simulink model "qbot2_sim_2020b"  (R2020b)
settings: Solver=FixedStepAuto  StartTime=0.0  StopTime=P.t_end  FixedStep=P.dt  RelTol=1e-3
InitFcn:
  | % load_qbot2_sim
StopFcn:
  | if (P.plotsim_flag)
  |     plot_sim(out, P)
  | end
settings Model: Creator=David L Olson  LastModifiedBy=divad

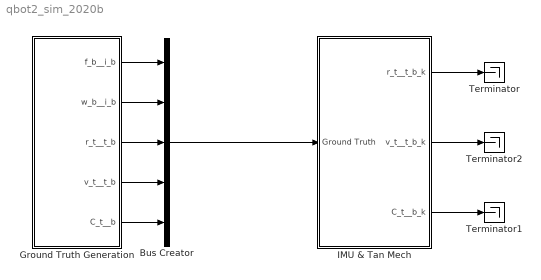
== system qbot2_sim_2020b ==
  Bus Creator : BusCreator  Inputs=5
  Ground Truth Generation : Subsystem
  IMU & Tan Mech : Subsystem
  Terminator : Terminator
  Terminator1 : Terminator
  Terminator2 : Terminator
  wires:
  Ground Truth Generation/1(f_b__i_b) -> Bus Creator/1
  Ground Truth Generation/2(w_b__i_b) -> Bus Creator/2
  Ground Truth Generation/3(r_t__t_b) -> Bus Creator/3
  Ground Truth Generation/4(v_t__t_b) -> Bus Creator/4
  Ground Truth Generation/5(C_t__b) -> Bus Creator/5
  Bus Creator/1 -> IMU & Tan Mech/1(Ground Truth)
  IMU & Tan Mech/1(r_t__t_b_k) -> Terminator/1
  IMU & Tan Mech/2(v_t__t_b_k) -> Terminator2/1
  IMU & Tan Mech/3(C_t__b_k) -> Terminator1/1

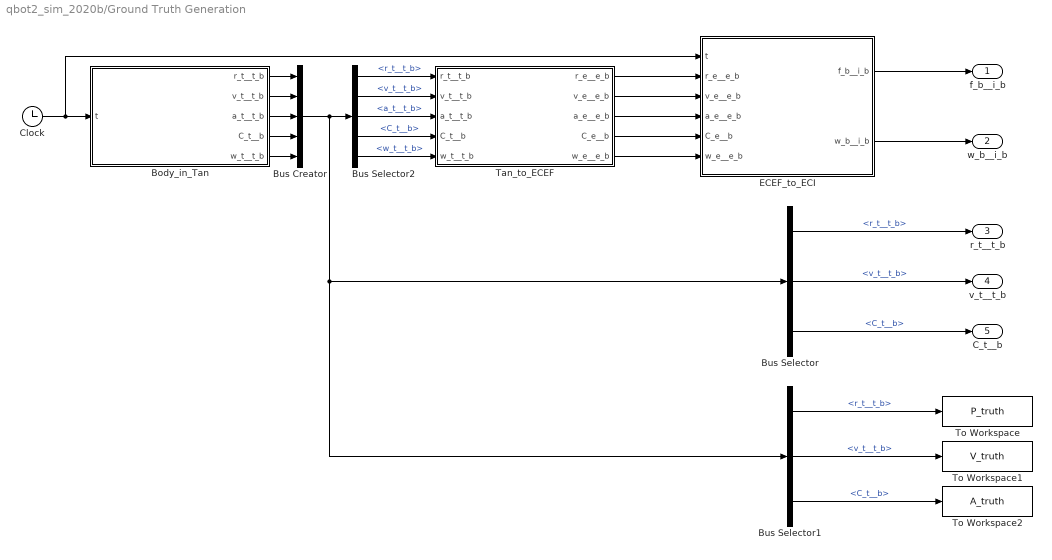
== system qbot2_sim_2020b/Ground Truth Generation ==
  Body_in_Tan : MATLAB Function  TreatAsAtomicUnit=on
  Bus Creator : BusCreator  Inputs=5
  Bus Selector : BusSelector  OutputSignals=r_t__t_b,v_t__t_b,C_t__b
  Bus Selector1 : BusSelector  OutputSignals=r_t__t_b,v_t__t_b,C_t__b
  Bus Selector2 : BusSelector  OutputSignals=r_t__t_b,v_t__t_b,a_t__t_b,C_t__b,w_t__t_b
  Clock : Clock
  ECEF_to_ECI : MATLAB Function  TreatAsAtomicUnit=on
  Tan_to_ECEF : MATLAB Function  TreatAsAtomicUnit=on
  To Workspace : ToWorkspace  VariableName=P_truth  SaveFormat=Timeseries  SampleTime=-1
  To Workspace1 : ToWorkspace  VariableName=V_truth  SaveFormat=Timeseries  SampleTime=-1
  To Workspace2 : ToWorkspace  VariableName=A_truth  SaveFormat=Timeseries  SampleTime=-1
  f_b__i_b : Outport
  w_b__i_b : Outport  Port=2
  r_t__t_b : Outport  Port=3
  v_t__t_b : Outport  Port=4
  C_t__b : Outport  Port=5
  wires:
  Clock/1 -> Body_in_Tan/1(t), ECEF_to_ECI/1(t)
  Tan_to_ECEF/1(r_e__e_b) -> ECEF_to_ECI/2(r_e__e_b)
  Tan_to_ECEF/3(a_e__e_b) -> ECEF_to_ECI/4(a_e__e_b)
  Tan_to_ECEF/2(v_e__e_b) -> ECEF_to_ECI/3(v_e__e_b)
  Tan_to_ECEF/4(C_e__b) -> ECEF_to_ECI/5(C_e__b)
  Tan_to_ECEF/5(w_e__e_b) -> ECEF_to_ECI/6(w_e__e_b)
  ECEF_to_ECI/2(w_b__i_b) -> w_b__i_b/1
  ECEF_to_ECI/1(f_b__i_b) -> f_b__i_b/1
  Body_in_Tan/1(r_t__t_b) -> Bus Creator/1
  Body_in_Tan/2(v_t__t_b) -> Bus Creator/2
  Body_in_Tan/3(a_t__t_b) -> Bus Creator/3
  Body_in_Tan/4(C_t__b) -> Bus Creator/4
  Body_in_Tan/5(w_t__t_b) -> Bus Creator/5
  Bus Creator/1 -> Bus Selector2/1, Bus Selector/1, Bus Selector1/1
  Bus Selector/1 -> r_t__t_b/1  "<r_t__t_b>"
  Bus Selector/2 -> v_t__t_b/1  "<v_t__t_b>"
  Bus Selector/3 -> C_t__b/1  "<C_t__b>"
  Bus Selector2/5 -> Tan_to_ECEF/5(w_t__t_b)  "<w_t__t_b>"
  Bus Selector2/4 -> Tan_to_ECEF/4(C_t__b)  "<C_t__b>"
  Bus Selector2/3 -> Tan_to_ECEF/3(a_t__t_b)  "<a_t__t_b>"
  Bus Selector2/2 -> Tan_to_ECEF/2(v_t__t_b)  "<v_t__t_b>"
  Bus Selector2/1 -> Tan_to_ECEF/1(r_t__t_b)  "<r_t__t_b>"
  Bus Selector1/2 -> To Workspace1/1  "<v_t__t_b>"
  Bus Selector1/1 -> To Workspace/1  "<r_t__t_b>"
  Bus Selector1/3 -> To Workspace2/1  "<C_t__b>"

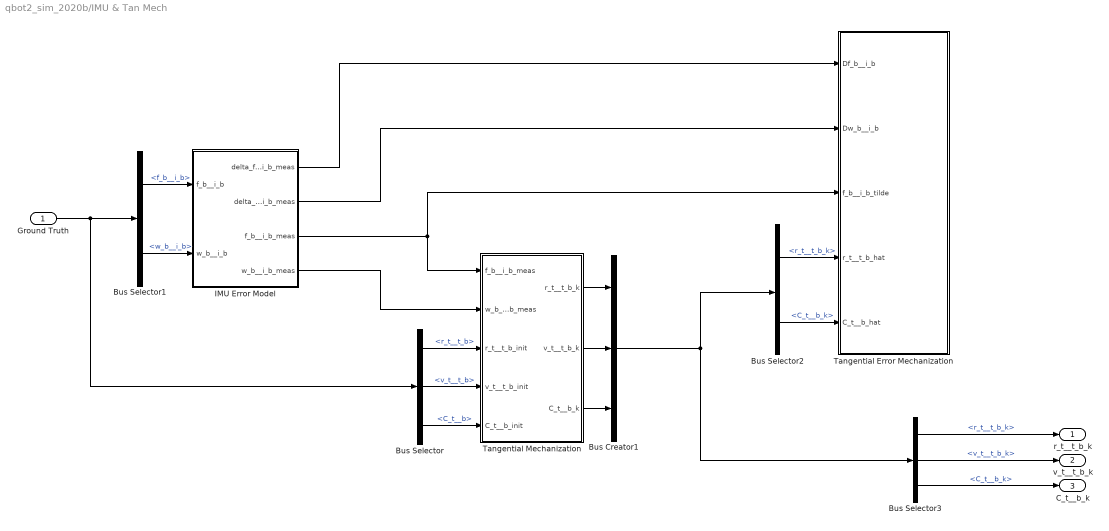
== system qbot2_sim_2020b/IMU & Tan Mech ==
  Ground Truth : Inport
  Bus Creator1 : BusCreator  Inputs=3
  Bus Selector : BusSelector  OutputSignals=r_t__t_b,v_t__t_b,C_t__b
  Bus Selector1 : BusSelector  OutputSignals=f_b__i_b,w_b__i_b
  Bus Selector2 : BusSelector  OutputSignals=r_t__t_b_k,C_t__b_k
  Bus Selector3 : BusSelector  OutputSignals=r_t__t_b_k,v_t__t_b_k,C_t__b_k
  IMU Error Model : Subsystem
  Tangential Error Mechanization : Subsystem
  Tangential Mechanization : Subsystem
  r_t__t_b_k : Outport
  v_t__t_b_k : Outport  Port=2
  C_t__b_k : Outport  Port=3
  wires:
  Bus Selector1/1 -> IMU Error Model/1(f_b__i_b)  "<f_b__i_b>"
  IMU Error Model/4(w_b__i_b_meas) -> Tangential Mechanization/2(w_b__i_b_meas)
  Tangential Mechanization/3(C_t__b_k) -> Bus Creator1/3
  IMU Error Model/1(delta_f_b__i_b_meas) -> Tangential Error Mechanization/1(Df_b__i_b)
  IMU Error Model/3(f_b__i_b_meas) -> Tangential Mechanization/1(f_b__i_b_meas), Tangential Error Mechanization/3(f_b__i_b_tilde)
  Bus Selector1/2 -> IMU Error Model/2(w_b__i_b)  "<w_b__i_b>"
  Tangential Mechanization/2(v_t__t_b_k) -> Bus Creator1/2
  IMU Error Model/2(delta_w_b__i_b_meas) -> Tangential Error Mechanization/2(Dw_b__i_b)
  Tangential Mechanization/1(r_t__t_b_k) -> Bus Creator1/1
  Bus Selector2/2 -> Tangential Error Mechanization/5(C_t__b_hat)  "<C_t__b_k>"
  Bus Selector/3 -> Tangential Mechanization/5(C_t__b_init)  "<C_t__b>"
  Bus Selector/2 -> Tangential Mechanization/4(v_t__t_b_init)  "<v_t__t_b>"
  Bus Creator1/1 -> Bus Selector2/1, Bus Selector3/1
  Ground Truth/1 -> Bus Selector1/1, Bus Selector/1
  Bus Selector3/2 -> v_t__t_b_k/1  "<v_t__t_b_k>"
  Bus Selector/1 -> Tangential Mechanization/3(r_t__t_b_init)  "<r_t__t_b>"
  Bus Selector2/1 -> Tangential Error Mechanization/4(r_t__t_b_hat)  "<r_t__t_b_k>"
  Bus Selector3/1 -> r_t__t_b_k/1  "<r_t__t_b_k>"
  Bus Selector3/3 -> C_t__b_k/1  "<C_t__b_k>"

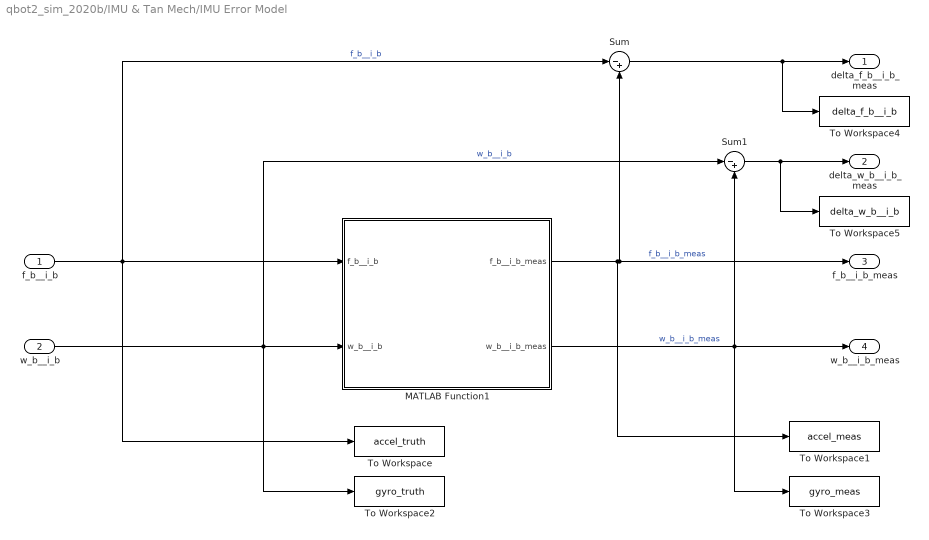
== system qbot2_sim_2020b/IMU & Tan Mech/IMU Error Model ==
  f_b__i_b : Inport
  w_b__i_b : Inport  Port=2
  MATLAB Function1 : MATLAB Function  TreatAsAtomicUnit=on
  Sum : Sum  Inputs=|-+
  Sum1 : Sum  Inputs=|-+
  To Workspace : ToWorkspace  VariableName=accel_truth  SaveFormat=Timeseries  SampleTime=-1
  To Workspace1 : ToWorkspace  VariableName=accel_meas  SaveFormat=Timeseries  SampleTime=-1
  To Workspace2 : ToWorkspace  VariableName=gyro_truth  SaveFormat=Timeseries  SampleTime=-1
  To Workspace3 : ToWorkspace  VariableName=gyro_meas  SaveFormat=Timeseries  SampleTime=-1
  To Workspace4 : ToWorkspace  VariableName=delta_f_b__i_b  SaveFormat=Timeseries  SampleTime=-1
  To Workspace5 : ToWorkspace  VariableName=delta_w_b__i_b  SaveFormat=Timeseries  SampleTime=-1
  delta_f_b__i_b_meas : Outport
  delta_w_b__i_b_meas : Outport  Port=2
  f_b__i_b_meas : Outport  Port=3
  w_b__i_b_meas : Outport  Port=4
  wires:
  f_b__i_b/1 -> To Workspace/1, Sum/1, MATLAB Function1/1(f_b__i_b)  "f_b__i_b"
  w_b__i_b/1 -> Sum1/1, To Workspace2/1, MATLAB Function1/2(w_b__i_b)  "w_b__i_b"
  MATLAB Function1/1(f_b__i_b_meas) -> f_b__i_b_meas/1, Sum/2, To Workspace1/1  "f_b__i_b_meas"
  MATLAB Function1/2(w_b__i_b_meas) -> Sum1/2, w_b__i_b_meas/1, To Workspace3/1  "w_b__i_b_meas"
  Sum1/1 -> To Workspace5/1, delta_w_b__i_b_meas/1
  Sum/1 -> To Workspace4/1, delta_f_b__i_b_meas/1

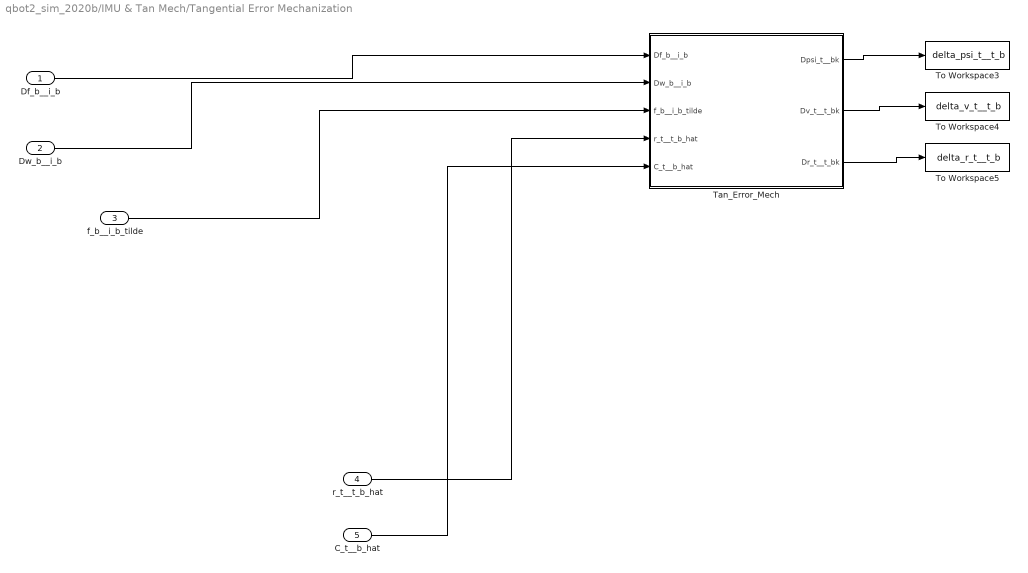
== system qbot2_sim_2020b/IMU & Tan Mech/Tangential Error Mechanization ==
  Df_b__i_b : Inport
  Dw_b__i_b : Inport  Port=2
  f_b__i_b_tilde : Inport  Port=3
  r_t__t_b_hat : Inport  Port=4
  C_t__b_hat : Inport  Port=5
  Tan_Error_Mech : MATLAB Function  TreatAsAtomicUnit=on
  To Workspace3 : ToWorkspace  VariableName=delta_psi_t__t_b  SaveFormat=Timeseries  SampleTime=-1
  To Workspace4 : ToWorkspace  VariableName=delta_v_t__t_b  SaveFormat=Timeseries  SampleTime=-1
  To Workspace5 : ToWorkspace  VariableName=delta_r_t__t_b  SaveFormat=Timeseries  SampleTime=-1
  wires:
  Tan_Error_Mech/2(Dv_t__t_bk) -> To Workspace4/1
  Tan_Error_Mech/1(Dpsi_t__bk) -> To Workspace3/1
  f_b__i_b_tilde/1 -> Tan_Error_Mech/3(f_b__i_b_tilde)
  r_t__t_b_hat/1 -> Tan_Error_Mech/4(r_t__t_b_hat)
  C_t__b_hat/1 -> Tan_Error_Mech/5(C_t__b_hat)
  Dw_b__i_b/1 -> Tan_Error_Mech/2(Dw_b__i_b)
  Tan_Error_Mech/3(Dr_t__t_bk) -> To Workspace5/1
  Df_b__i_b/1 -> Tan_Error_Mech/1(Df_b__i_b)

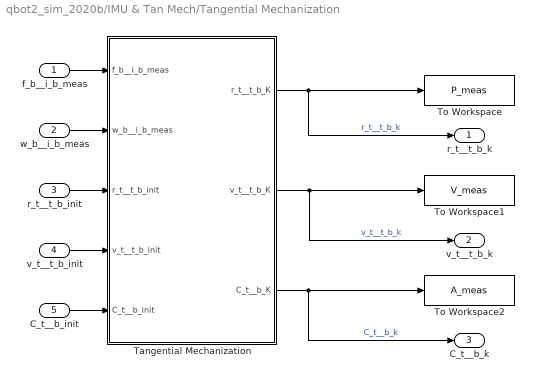
== system qbot2_sim_2020b/IMU & Tan Mech/Tangential Mechanization ==
  f_b__i_b_meas : Inport
  w_b__i_b_meas : Inport  Port=2
  r_t__t_b_init : Inport  Port=3
  v_t__t_b_init : Inport  Port=4
  C_t__b_init : Inport  Port=5
  Tangential Mechanization : MATLAB Function  TreatAsAtomicUnit=on
  To Workspace : ToWorkspace  VariableName=P_meas  SaveFormat=Timeseries  SampleTime=-1
  To Workspace1 : ToWorkspace  VariableName=V_meas  SaveFormat=Timeseries  SampleTime=-1
  To Workspace2 : ToWorkspace  VariableName=A_meas  SaveFormat=Timeseries  SampleTime=-1
  r_t__t_b_k : Outport
  v_t__t_b_k : Outport  Port=2
  C_t__b_k : Outport  Port=3
  wires:
  Tangential Mechanization/3(C_t__b_K) -> C_t__b_k/1, To Workspace2/1  "C_t__b_k"
  f_b__i_b_meas/1 -> Tangential Mechanization/1(f_b__i_b_meas)
  Tangential Mechanization/1(r_t__t_b_K) -> r_t__t_b_k/1, To Workspace/1  "r_t__t_b_k"
  C_t__b_init/1 -> Tangential Mechanization/5(C_t__b_init)
  v_t__t_b_init/1 -> Tangential Mechanization/4(v_t__t_b_init)
  r_t__t_b_init/1 -> Tangential Mechanization/3(r_t__t_b_init)
  w_b__i_b_meas/1 -> Tangential Mechanization/2(w_b__i_b_meas)
  Tangential Mechanization/2(v_t__t_b_K) -> v_t__t_b_k/1, To Workspace1/1  "v_t__t_b_k"

== matlab function qbot2_sim_2020b/Ground Truth Generation/Body_in_Tan ==
  data: r_t__t_b output; v_t__t_b output; a_t__t_b output; C_t__b output; w_t__t_b output; t input; P parameter
function [r_t__t_b, v_t__t_b, a_t__t_b, C_t__b, w_t__t_b] = ...
                                           Body_in_Tan(t, P)
                                       
%% QBOT2_TAN_GROUND_TRUTH_GEN Generates the motion of the body of the Qbot2
%wrt to the tangential frame.  

% Creating figure eight loop pattern for Qbot2.  The motion is unrealistic
% for the robot itself, however for now this verify all equations have been
% implemented correctly in all 3 dimensions.  

persistent init_flag C_t__b_old

% Extra Steps for MATLAB parser to properly function
if (isempty(init_flag))
    init_flag = 0;
    C_t__b_old = eye(3);
end

% {t} frame is set Noth East Down (NED)
% Position of {b} wrt {t} in the {t} frame (m) 
a = 0.25;
r_t__t_b = [0; 0; 0];
        
% Velocity of {b} wrt {t} in the {t} frame (m/s)
v_t__t_b = [0; 0; 0];
        
% Acceleration of {b} wrt {t} in the {t} frame (m/s^2)
a_t__t_b = [0; 0; 0];

w_t__t_b = zeros(3,1);

C_t__b = eye(3);

% % Figure Eight Parameters
% T = P.t_end;   % Period
% f = 1/T;       % Frequency
% w = 4*pi*f;    % Natural Frequency
% 
% % Figure Eight Amplitudes in {t} frame
% Ax = 1;
% Ay = 0.55;
% Az = 0.025;
% 
% % {t} frame is set Noth East Down (NED)
% % Position of {b} wrt {t} in the {t} frame (m) 
% r_t__t_b = [      Ax*sin(w*t); ...
%                  -Ay*sin((w/2)*t); ...
%              Az - Az*cos((2*w)*t)];
%         
% % Velocity of {b} wrt {t} in the {t} frame (m/s)
% v_t__t_b = [    w * Ax*cos(w*t); ...
%            -(w/2) * Ay*cos((w/2)*t); ...
%             (2*w) * Az*sin((2*w)*t)];
%         
% % Acceleration of {b} wrt {t} in the {t} frame (m/s^2)
% a_t__t_b = [   -w^2 * Ax*sin(w*t); ...
%             (w/2)^2 * Ay*sin((w/2)*t); ...
%             (2*w)^2 * Az*cos((2*w)*t)];
% %          
% % Orientation of {b} wrt {t} in the {t} frame (forward-right-down frame)
% x_axis = v_t__t_b / norm(v_t__t_b); % Due to plant dynamics
% 
% % Determine Pitch and Yaw in {t} frame
% roll = 0;
% pitch = -asin(x_axis(3));
% yaw = atan2(x_axis(2), x_axis(1));
% C_t__b_temp = ypr2dcm(yaw, pitch, roll);
% 
% % Rotate a_t__t_b into {b} frame, compare w/ gravity vector for Roll
% a_b__t_b_temp = C_t__b_temp' * a_t__t_b;
% roll = atan2(a_b__t_b_temp(2), 10);
% C_t__b = ypr2dcm(yaw, pitch, roll); 
% 
% if (init_flag == 0) % first time entering function
%     w_t__t_b = [0; 0; 0];
%     init_flag = 1;
%     C_t__b_old = eye(3);
% else % Be sure to ask about initial method of what went wrong
%     delta_C = C_t__b * C_t__b_old';
%     w_t__t_b = dcm2k(delta_C) / P.dt;
% end

% Store value of C_t__b for next iteration
C_t__b_old = C_t__b;

end

== matlab function qbot2_sim_2020b/IMU & Tan Mech/Tangential Mechanization/Tangential Mechanization ==
  data: f_b__i_b_meas input; w_b__i_b_meas input; r_t__t_b_init input; v_t__t_b_init input; C_t__b_init input; r_t__t_b_K output; P parameter; v_t__t_b_K output; C_t__b_K output
function [r_t__t_b_K, v_t__t_b_K, C_t__b_K] = Tan_Mech(f_b__i_b_meas, w_b__i_b_meas, r_t__t_b_init, v_t__t_b_init, C_t__b_init, P)

%% Tan_Mech
% Provides tangential mechanization for kinematic states position, velocity
% and attitude (PVA).  It does this solely based on accel and gyro
% measurements, which come from the IMU block.  The first time step is
% initialized from the ground truth block.  

persistent r_t__t_b_K_1 v_t__t_b_K_1 C_t__b_K_1 g_t__b

% Initialize on First Time Step
if (isempty(r_t__t_b_K_1))
    
    % Use "truth" to initialize on first time step
    r_t__t_b_K = r_t__t_b_init;
    v_t__t_b_K = v_t__t_b_init;
    C_t__b_K   = C_t__b_init;
    
    % Store current values as old values for next iteration
    r_t__t_b_K_1 = r_t__t_b_K;
    v_t__t_b_K_1 = v_t__t_b_K;
    C_t__b_K_1   = C_t__b_K;
    
    % Calculate and store the vector g_t__b
    r_e__e_b = P.r_e__e_t + P.C_e__t*r_t__t_b_init;         % Compute r_e__e_b
    [L_b, lambda_b, h_b] = xyz2llh(r_e__e_b, P);            % Compute the lat, lon, and height
    g_n__b = [0; 0; gravity(L_b, h_b, P)];                  % Compute the acceleration due to gravity
    C_e__n = Lat_Lon_2C_e__n(L_b, lambda_b);                % Compute C_e__n
    g_e__b = C_e__n * g_n__b;                               % Compute the gravity of the body in the {e} frame
    g_t__b = P.C_e__t' * g_e__b;                            % Compute the gravity of the body in the {t} frame 
    
    
    
% Every Other Time Step
else
    
    % C_t__b Rotation Matrix Update 
    if (P.fidelity == 0) % Low Fidelity Method
         
        Ohm_b__i_b_meas = vec2ss(w_b__i_b_meas);
        
        C_t__b_K = C_t__b_K_1*(eye(3) + Ohm_b__i_b_meas*P.dt) - ...
                                              P.Ohm_t__i_e*C_t__b_K_1*P.dt;
                                        
    elseif (P.fidelity == 1) % High Fidelity Method
        
        w_t__t_b = C_t__b_K_1*w_b__i_b_meas - P.C_e__t'*P.w_i__i_e;
        
        % Catch for when w_t__t_b is super super small
        if (norm(w_t__t_b) < 1e-6)
            C_t__b_K = C_t__b_K_1;
        else
            C_t__b_K = Rodrigues_k(w_t__t_b * P.dt) * C_t__b_K_1;
        end
        
    end
    
    % f_t__i_b Specific Force Update
    f_t__i_b = C_t__b_K * f_b__i_b_meas;
    
    % a_t__t_b Acceleration Vector Update
    
    a_t__t_b = f_t__i_b + g_t__b - 2*P.Ohm_t__i_e*v_t__t_b_K_1;
    
    % v_t__t_b Velocity Vector Update
    v_t__t_b_K = v_t__t_b_K_1 + a_t__t_b*P.dt;
    
    % r_t__t_b Position Vector Update
    r_t__t_b_K = r_t__t_b_K_1 + v_t__t_b_K_1*P.dt + a_t__t_b*((P.dt^2)/2);
    
    % Store new PVA as old PVA
    r_t__t_b_K_1 = r_t__t_b_K;
    v_t__t_b_K_1 = v_t__t_b_K;
    C_t__b_K_1   = C_t__b_K;
    
end

== matlab function qbot2_sim_2020b/Ground Truth Generation/Tan_to_ECEF ==
  data: r_t__t_b input; v_t__t_b input; a_t__t_b input; C_t__b input; w_t__t_b input; r_e__e_b output; v_e__e_b output; a_e__e_b output; C_e__b output; w_e__e_b output; P parameter
function [r_e__e_b, v_e__e_b, a_e__e_b, C_e__b, w_e__e_b] = ...
             Tan_to_ECEF(r_t__t_b, v_t__t_b, a_t__t_b, C_t__b, w_t__t_b, P)
         
%% Tan_to_ECEF 
% Transfroms motion in the {t} frame into the {e} frame.  The 'P' structure
% contains data relevant to making the {t}->{e} transforms specifically to
% my house in Minot ND.  (1124 9th St NW, Minot ND 58703)

% Position of the {b} frame wrt the {e} frame resolved in {e} (m)
r_e__e_b = P.r_e__e_t + P.C_e__t*r_t__t_b;

% Velocity of the {b} frame wrt the {e} frame resolved in {e} (m/s)
v_e__e_b = P.C_e__t*v_t__t_b;
       
% Acceleration of the b-frame wrt the e-frame resolved in {e} (m/s^2)
a_e__e_b = P.C_e__t*a_t__t_b;
        
%Attitude of the {b} frame wrt the {e} frame (unitless)
C_e__b = P.C_e__t*C_t__b;         

% Angular velocity of the {b} frame wrt the {e} frame resolved in {e} (rad/s)
w_e__e_b = P.C_e__t*w_t__t_b;

== matlab function qbot2_sim_2020b/Ground Truth Generation/ECEF_to_ECI ==
  data: t input; f_b__i_b output; r_e__e_b input; v_e__e_b input; a_e__e_b input; C_e__b input; w_e__e_b input; w_b__i_b output; P parameter
function [f_b__i_b, w_b__i_b] = ...
          ECEF_to_ECI(t, r_e__e_b, v_e__e_b, a_e__e_b, C_e__b, w_e__e_b, P)

%% ECEF to ECI
% Transforms motion from the ECEF frame to the ECI frame
% This assumes the simulation always starts at 0000z

% Calculate g_n__b only once, since area of travel is so small
persistent g_e__b

if (isempty(g_e__b))
    [L_b, lambda_b, h_b] = xyz2llh(r_e__e_b, P);
    g_n__b = [0; 0; gravity(L_b, h_b, P)];
    C_e__n = Lat_Lon_2C_e__n(L_b, lambda_b);
    g_e__b = C_e__n * g_n__b;
end

% Generate earth's rotation from {i} frame to {e} frame
theta_ie = P.w_ie * t + 0;

C_i__e = [cos(theta_ie), -sin(theta_ie), 0; ...
          sin(theta_ie),  cos(theta_ie), 0; ...
          0,              0,             1];    
      
% Position of {b} frame wrt {t} frame resolved in {i} frame (m)
r_i__i_b = C_i__e*r_e__e_b;

% Velocity of {b} frame wrt {i} frame resolved in {i} frame (m/s)
v_i__i_b = C_i__e*v_e__e_b + P.Ohm_i__i_e*C_i__e*r_e__e_b;

% Acceleration of {b} frame wrt {i} frame resolved in {i} frame (m/s^2)
a_i__i_b = C_i__e*a_e__e_b + 2*P.Ohm_i__i_e*C_i__e*v_e__e_b + ...
                                 P.Ohm_i__i_e*P.Ohm_i__i_e*C_i__e*r_e__e_b;
                                       
% Attitude of {b} frame wrt to {i} frame
C_i__b = C_i__e*C_e__b;

% Angular Velocity: Ideal Gyro Measurements
w_b__i_b = C_i__b' * (P.w_i__i_e + C_i__e*w_e__e_b);

% Specific Force: Ideal Accel Measurements
f_b__i_b = C_i__b' * (a_i__i_b - C_i__e*g_e__b - ...
                                       P.Ohm_i__i_e*P.Ohm_i__i_e*r_i__i_b);
                                   
% % Dummy Action for Debugging
% dummy = 1;

== matlab function qbot2_sim_2020b/IMU & Tan Mech/IMU Error Model/MATLAB Function1 ==
  data: f_b__i_b input; f_b__i_b_meas output; w_b__i_b input; w_b__i_b_meas output; P parameter
function [f_b__i_b_meas, w_b__i_b_meas] = IMU(f_b__i_b, w_b__i_b, P)
% IMU models the IMU error characteristics, taking truth as the input and
% outputs measurements that are subject to errors.  These errors stem from
% data obtained from the VN200 used for hardware implementation.  

%% Function Initializatoin

persistent b_g_BI b_a_BI

if isempty(b_g_BI)
    b_g_BI = [0; 0; 0];
    b_a_BI = [0; 0; 0];
end


%% Define P

%  General P
dt = P.dt;
Fs = P.Fs;
I3 = eye(3);

% Gyro Related Terms
b_g_BI_sigma_n = P.gyro.BI.sigma_n;  % Bias - White Noise driving the Bias Instability 1-sigma (rad/s)

tau_g        = P.gyro.BI.correlation_time;  % Correlation time for the bias instability (sec)
b_g_FB       = P.gyro.b_g_FB;               % Bias - Fixed Bias term (rad/s)

sigma_ARW   = P.gyro.sigma_ARW;             % Standard deviation of white noise due to ARW (rad/s)
M_g         = P.gyro.M_g;                   % The combined Gyro Misalignment/Scale-Factor matrix
G_g         = P.gyro.G_g;                   % The gyro G-sensitivity matrix (rad/sec/g)

 % Accel related terms   
b_a_BI_sigma_n = P.accel.BI.sigma_n;        % Bias - White noise driving the Bias Instability 1-sigma (m/s^2)

tau_a        = P.accel.BI.correlation_time; % Correlation time for the bias instability (sec)
b_a_FB       = P.accel.b_a_FB;              % Bias - Fixed Bias term (m/s^2)

sigma_VRW   = P.accel.sigma_VRW;            % Standard deviation of white noise due to VRW (m/s^2)
M_a         = P.accel.M_a;                  % The combined Gyro Misalignment/Scale-Factor matrix    

%++++++++++++++++++++++++++++++++++++++++++++++++++++++++++++++++++++++++++
% Gyro Model:
%++++++++++++++++++++++++++++++++++++++++++++++++++++++++++++++++++++++++++

% Bias terms
b_g_BS = P.gyro.b_g_BS;                                        % Bias - Bias Stability Bias term (rad/s)
b_g_BI = exp(-dt/tau_g) * b_g_BI + randn(3,1).*b_g_BI_sigma_n; % Bias - Markov Bias Instability Bias term (rad/s)
b_g = b_g_BI + b_g_FB + b_g_BS;                                % All three bias terms (rad/s)

% Noise terms
w_g = sigma_ARW .* randn(3,1);                                 % Gyro noise (rad/sec)

% Including all of the error terms
w_b__i_b_meas = b_g + (I3 + M_g) * w_b__i_b + G_g * f_b__i_b + w_g;

%++++++++++++++++++++++++++++++++++++++++++++++++++++++++++++++++++++++++++
% Accelerometer Model
%++++++++++++++++++++++++++++++++++++++++++++++++++++++++++++++++++++++++++

% Bias terms
b_a_BS = P.accel.b_a_BS;                                       % Bias - Bias Stability Bias term (m/s^2)
b_a_BI = exp(-dt/tau_a) * b_a_BI + randn(3,1).*b_a_BI_sigma_n; % Bias - Markov Bias Instability Bias term (m/s^2)
b_a = b_a_BI + b_a_FB + b_a_BS;                                % All three bias terms (m/s^2)

% Noise terms
w_a = sigma_VRW .* randn(3,1);                                 % Accelerometer noise (in m/s^2)

% Including all of the error terms
f_b__i_b_meas = b_a + (I3 + M_a) * f_b__i_b + w_a;

== matlab function qbot2_sim_2020b/IMU & Tan Mech/Tangential Error Mechanization/Tan_Error_Mech ==
  data: Df_b__i_b input; Dpsi_t__bk output; Dw_b__i_b input; f_b__i_b_tilde input; r_t__t_b_hat input; C_t__b_hat input; Dv_t__t_bk output; Dr_t__t_bk output; P parameter
function [Dpsi_t__bk, Dv_t__t_bk, Dr_t__t_bk] = Tan_Error_mech(Df_b__i_b, Dw_b__i_b, f_b__i_b_tilde, r_t__t_b_hat, C_t__b_hat, P)
%#codegen
% FUNCTION DESCRIPTION:
%   Implements the Tangential Frame Error-Mechanization
%
% INPUTS:
%   Df_b__i_b       = Error in Current Accel measurements (m/s^2)
%   Dw_b__i_b       = Error in Current gyro measurements (rad/s)
%   f_b__i_b_tilde  = Current Accel measurements (m/s^2)
%   r_t__t_b_hat    = Position estimate from TAN mech (meters)
%   C_t__b_hat      = Attitude estimate from TAN mech
%
% OUTPUTS:
%   Dpsi_t__bk      = Delta psi      vector (rad)
%   Dv_t__t_bk      = Delta velocity vector (meters/sec)
%   Dr_t__t_bk      = Delta position vector (meters)
%
%  Reference:  EE 440 Lecture notes:
%       lectures 29 & 30
%  NOTES:
%    Groves Chap 14 Section 2

persistent Delta_PVAk_1

dt         = P.dt;          % Time step (sec)
I3         = eye(3);                % 3X3 Identity matrix
Ohm_i__i_e = P.Ohm_i__i_e;  % Skew symmetric version of w_i__i_e (rad/s)
C_e__t     = P.C_e__t;   	% Attitude of t-frame wrt e-frame (a constant matrix)
C_t__e     = C_e__t';
r_e__e_t   = P.r_e__e_t;    % Position of org of t-frame wrt e-frame resolved in e-frame
   
if isempty(Delta_PVAk_1)    
    Delta_PVAk_1  = zeros(9,1);     % Initialize Delta_PVA(k-1)
    Delta_PVAk    = zeros(9,1);     % Initialize Delta_PVA(k-1)
else
    Delta_PVAk = eye(9);
%% Build the F matrix: See lecture 29 slide 7
    O3 = zeros(3,3);
% First row:
    Ohm_t__i_e = C_t__e * Ohm_i__i_e * C_e__t;  % Earth rate in the t-frame

% Second row:
    F21 = -vec2ss(C_t__b_hat * f_b__i_b_tilde); % Vector to Skew-Symmetric
  % Now build F23
    r_e__e_b_hat = r_e__e_t + C_e__t * r_t__t_b_hat;
    [L_b_hat, lambda_b_hat, h_b_hat] = xyz2llh(r_e__e_b_hat, P);
    gamma_e__i_b = gamma__i_b(r_e__e_b_hat, P);
    r_e__e_S = Geo_Radius(L_b_hat, P);
 
    F23 = -C_t__e * 2 * gamma_e__i_b * r_e__e_b_hat' / (r_e__e_S * norm(r_e__e_b_hat)) * C_e__t;
     
    F = [ -Ohm_t__i_e   ,  O3               , O3
           F21          , -2* Ohm_t__i_e    , F23
           O3           ,  I3               , O3];

%% Build the B matrix: See lecture 29 slide 7
    B = [O3         , C_t__b_hat
         C_t__b_hat , O3
         O3         , O3];

%% Transform Eqns from continuous-time to discrete-time: Lecture 30 slides 9-10
    Phi = eye(9) + F*dt;                % Estimate of exp(F dt) = I + F dt + F^2 dt^2 /2! + ...
	G  = (eye(9)*dt + F*dt^2/2) * B;    % Estimate of G = A^-1 (exp(F dt) - I ) B = (I dt + F dt^2 /2! + ...) B

    Delta_PVAk = Phi*Delta_PVAk_1 + G * [Df_b__i_b; Dw_b__i_b];

    Delta_PVAk_1 = Delta_PVAk;          % Store Delta_PVA(k) into Delta_PVA(k-1) for next iteration
end

Dpsi_t__bk = Delta_PVAk(1:3,1);   % Extract the Attitude errror terms
Dv_t__t_bk = Delta_PVAk(4:6,1);   % Extract the velocity errror terms
Dr_t__t_bk = Delta_PVAk(7:9,1);   % Extract the position errror terms
end     % End of function
